simulink model "PurePursuit"  (R2023b)
settings: Solver=FixedStepAuto  StartTime=0.0  StopTime=inf  FixedStep=0.0018  RelTol=1e-3
undefined symbols (not defined in the file): angular, linear, waypoints
libraries: ros2lib x3, robotalgslib x1
settings Model: Creator=alogo  LastModifiedBy=alogo

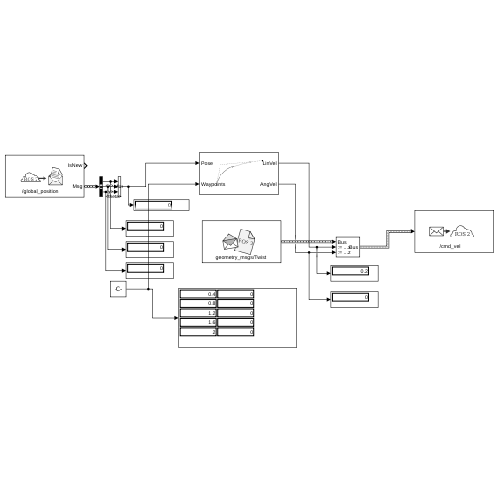
[thumbnail: Simulink's stored preview of the top-level diagram]
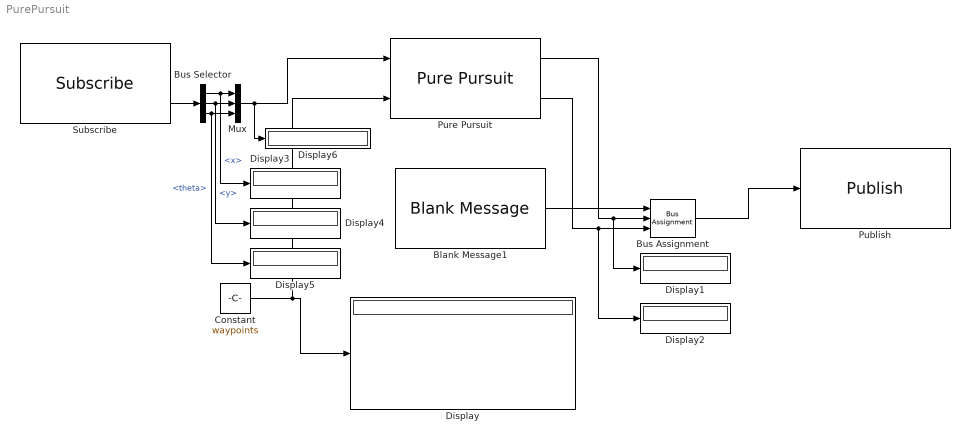
== system PurePursuit ==
  Blank Message1 : ros2lib/Blank Message  messageClass=Message  entityType=geometry_msgs/Twist  messageType=geometry_msgs/Twist  SampleTime=inf
  Bus Assignment : BusAssignment  AssignedSignals=linear.x,angular.z
  Bus Selector : BusSelector  OutputSignals=x,y,theta
  Constant : Constant  Value=waypoints
  Display{,1..6} (7 alike) : Display
  Mux : Mux  Inputs=3
  Publish : ros2lib/Publish  topicSource=Select from ROS network  topic=/cmd_vel  messageType=geometry_msgs/Twist  QOSHistory=Keep last  QOSDepth=1  QOSReliability=Best effort  QOSDurability=Volatile
  Pure Pursuit : robotalgslib/Pure Pursuit  DesiredLinearVelocity=0.2  MaxAngularVelocity=0.1  LookaheadDistance=1.0  TargetDirPort=off  SimulateUsing=Code generation
      settings: LibrarySourceBlock=robotmobilelib/Pure Pursuit
  Subscribe : ros2lib/Subscribe  topicSource=Select from ROS network  topic=/global_position  messageType=geometry_msgs/Pose2D  sampleTime=-1  QOSHistory=Keep last  QOSDepth=1  QOSReliability=Best effort  QOSDurability=Volatile
  wires:
  Subscribe/2 -> Bus Selector/1
  Bus Selector/1 -> Display3/1, Mux/1  "<x>"
  Bus Selector/2 -> Display4/1, Mux/2  "<y>"
  Bus Selector/3 -> Display5/1, Mux/3  "<theta>"
  Mux/1 -> Display6/1, Pure Pursuit/1
  Blank Message1/1 -> Bus Assignment/1
  Bus Assignment/1 -> Publish/1
  Pure Pursuit/1 -> Display1/1, Bus Assignment/2
  Pure Pursuit/2 -> Display2/1, Bus Assignment/3
  Constant/1 -> Display/1, Pure Pursuit/2
